simulink model "speechCommandRecognition"  (R2021a)
settings: Solver=FixedStepDiscrete  StartTime=0.0  StopTime=inf  RelTol=1e-3
InitFcn:
  | % Specify the audio sampling rate and classification rate in Hz and create
  | % an audio device reader that can read audio from your microphone.
  | fs = 16e3;
  | classificationRate = 10;
  | epsil = 1e-6;
  | numBands = 40;
  | 
  | % Audio device samples per frame
  | samplesPerFrame = floor(fs/classificationRate);
  | 
  | % Specify frameDuration and hopDuration for the melSpectrogram (in seconds)
  | frameDuration = 0.025;
  | hopDuration = 0.01;
  | 
  | % Frame and hop length for melSpectrogram in samples
  | frameLength = frameDuration*fs;
  | hopLength = hopDuration*fs;
  | 
  | % Spectrogram width (in time)
  | specWidthTime = 1 * fs;
  | 
  | % Spectrogram width (in samples)
  | specWidth = floor((specWidthTime-frameLength) / hopLength) + 1;
libraries: dspvision x3, audiosources x1, deeplib x1, simulink x1
settings Model: Creator=The MathWorks, Inc.  LastModifiedBy=The MathWorks, Inc.
settings SolverCC: AlgebraicLoopSolver=TrustRegion  AutoInsertRateTranBlk=on
settings DataIOCC: LimitDataPoints=on  SaveOutput=off  SignalLogging=off  SaveTime=off
settings OptimizationCC: LifeSpan=inf  SimCompilerOptimization=on
settings DebuggingCC: AlgebraicLoopMsg=error  SingleTaskRateTransMsg=error  IntegerOverflowMsg=none  AllowSymbolicDim=off  SFUnexpectedBacktrackingDiag=warning  SFNoUnconditionalDefaultTransitionDiag=warning  SFExecutionAtInitializationDiag=none  SFMachineParentedDataDiag=warning  IntegerSaturationMsg=none  ArithmeticOperatorsInVariantConditions=warning
settings SFSimCC: SimCtrlC=off  SimUseLocalCustomCode=off  CustomCodeUndefinedFunction=UseInterfaceOnly
settings RTWCC: RTWUseLocalCustomCode=off
settings CodeAppCC: StateflowObjectComments=on
settings GRTTargetCC: TargetLangStandard=C89/C90 (ANSI)
settings ConfigComp: CovMetricSettings=dw  CovSaveCumulativeToWorkspaceVar=on  CovSaveSingleToWorkspaceVar=on  CovExternalEMLEnable=off  CovSFcnEnable=off

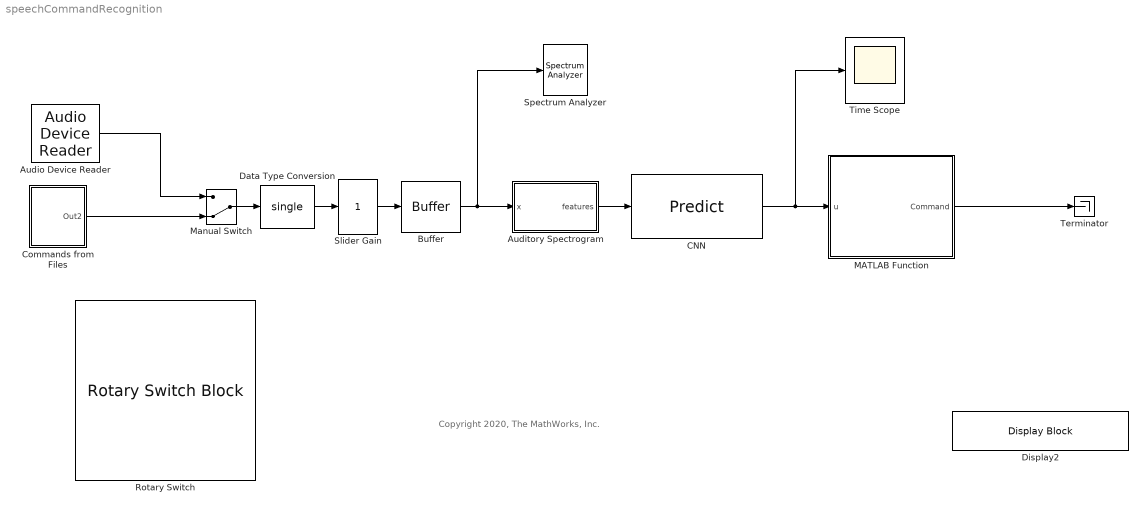
== system speechCommandRecognition ==
  note: Copyright 2020, The MathWorks, Inc.
  Audio Device Reader : audiosources/Audio Device Reader  Driver=CoreAudio  Device=No audio input device detected  SampleRate=fs  NumChannels=1  SamplesPerFrame=samplesPerFrame  BitDepth=16-bit integer  NumBuffers=10  DefaultInputChannelMapping=on  InputChannelMapping=1:2  OutputNumOverrunSamples=off  OutputDataType=double  DriverIdx=5  DeviceWarnFlag=''
      settings: SourceProductBaseCode=AU
  Auditory Spectrogram : MATLAB Function  TreatAsAtomicUnit=on
  Buffer : Buffer  N=fs  V=fs - samplesPerFrame  OutputFrames=off
  CNN : deeplib/Predict  Network=Network from MAT-file  NetworkFunction=squeezenet  NetworkFilePath=commandNet.mat  MiniBatchSize=1  InputDataFormats={ '', '' }  Predictions=off  Activations={ 'softmax' }  ForceInterpretedSim=off  EnableDLNetwork=off
      settings: SourceProductBaseCode=NN
  Commands from Files : Subsystem
  Data Type Conversion : DataTypeConversion  OutDataTypeStr=single
  Display2 : DisplayBlock  LabelPosition=Hide  Format=short
  MATLAB Function : MATLAB Function  TreatAsAtomicUnit=on
  Manual Switch : ManualSwitch  CurrentSetting=0
  Rotary Switch : RotarySwitchBlock
      settings: Values={{'Go', 'Yes', 'Stop'}, [1 2 3]}
  Slider Gain : simulink/Math Operations/Slider Gain  gain=1  low=0  high=30
  Spectrum Analyzer : SpectrumAnalyzer
  Terminator : Terminator
  Time Scope : Scope
  wires:
  Manual Switch/1 -> Data Type Conversion/1
  MATLAB Function/1(Command) -> Terminator/1
  Auditory Spectrogram/1(features) -> CNN/1
  Slider Gain/1 -> Buffer/1
  CNN/1 -> MATLAB Function/1(u), Time Scope/1
  Buffer/1 -> Auditory Spectrogram/1(x), Spectrum Analyzer/1
  Data Type Conversion/1 -> Slider Gain/1
  Commands from Files/1(Out2) -> Manual Switch/2
  Audio Device Reader/1 -> Manual Switch/1

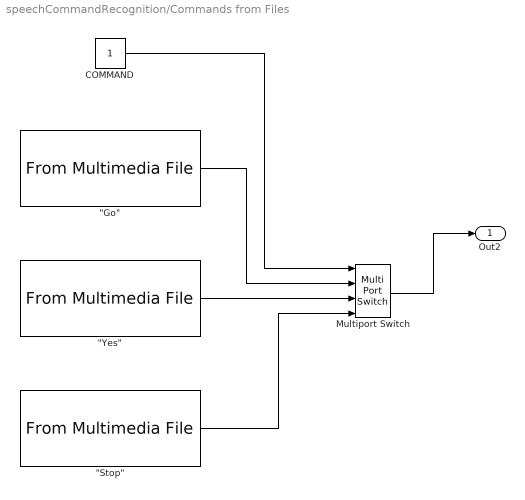
== system speechCommandRecognition/Commands from Files ==
  " \"Stop\"" : dspvision/From Multimedia File  inputFilename=stopCommand.flac  readRange=[1 Inf]  loop=on  numPlays=inf  outputStreams=Audio only  videoDataType=single  audioDataType=double  inheritSampleTime=on  userDefinedSampleTime=1/30  noAudioOutput=off  isIntensityVideo=off  fourcc=RGB  colorVideoFormat=Separate color signals  outputEOF=off  dataOrg=Column-major  audioFrameSize=samplesPerFrame  computeAudioFrameSize=off  outSamplingMode=Sample based
  "\"Go\"" : dspvision/From Multimedia File  inputFilename=goCommand.flac  readRange=[1 Inf]  loop=on  numPlays=inf  outputStreams=Audio only  videoDataType=single  audioDataType=double  inheritSampleTime=on  userDefinedSampleTime=1/30  noAudioOutput=off  isIntensityVideo=off  fourcc=RGB  colorVideoFormat=Separate color signals  outputEOF=off  dataOrg=Column-major  audioFrameSize=samplesPerFrame  computeAudioFrameSize=off  outSamplingMode=Sample based
  "\"Yes\"" : dspvision/From Multimedia File  inputFilename=yesCommand.flac  readRange=[1 Inf]  loop=on  numPlays=inf  outputStreams=Audio only  videoDataType=single  audioDataType=double  inheritSampleTime=on  userDefinedSampleTime=1/30  noAudioOutput=off  isIntensityVideo=off  fourcc=RGB  colorVideoFormat=Separate color signals  outputEOF=off  dataOrg=Column-major  audioFrameSize=samplesPerFrame  computeAudioFrameSize=off  outSamplingMode=Sample based
  COMMAND : Constant
  Multiport Switch : MultiPortSwitch
  Out2 : Outport
  wires:
  "\"Yes\""/1 -> Multiport Switch/3
  " \"Stop\""/1 -> Multiport Switch/4
  Multiport Switch/1 -> Out2/1
  "\"Go\""/1 -> Multiport Switch/2
  COMMAND/1 -> Multiport Switch/1

== matlab function speechCommandRecognition/MATLAB Function ==
  data: u input; classificationRate parameter; Command output size=[1 1]
function Command = postProcess(u,classificationRate)

    persistent YBuffer probBuffer
    
    if(isempty(YBuffer))
        YBuffer = ones(classificationRate,1);
        probBuffer = zeros([numel(u),round(classificationRate/2)]);
        prevCommand = SpeechCommands(0);
    end
    
    % Input u is array of 12 probability values (which word was most likely
    % to be spoken)

    % Find index of array with highest probability and enumerate to our
    % word
    [~,YPredicted] = max(u);
    
    % Add to buffers
    YBuffer(1:end-1)= YBuffer(2:end);
    YBuffer(end) = YPredicted;
    probBuffer(:,1:end-1) = probBuffer(:,2:end);
    probBuffer(:,end) = u;
    
    % Now do the actual command detection by performing a very simple
    % thresholding operation. Declare a detection and display it 
    % if all of the following hold:
    % 1) The most common label is not |background|.
    % 2) At least |countThreshold| of the latest frame labels agree.
    % 3) The maximum predicted probability of the predicted label is at
    % least |probThreshold|. Otherwise, do not declare a detection.

    [YMode,count] = mode(YBuffer,1);
    countThreshold = ceil(classificationRate*0.2);
    maxProb = max(probBuffer(YMode,:));
    probThreshold = 0.5;

    if (count > countThreshold && maxProb > probThreshold && YMode ~= SpeechCommands.Background)
        Command = SpeechCommands(YMode);
        prevCommand = Command;
    else
        Command = SpeechCommands(0);
    end
    
end

== matlab function speechCommandRecognition/Auditory Spectrogram ==
  data: x input size=[specWidthTime 1]; features output size=[98 50]
function features = fcn(x)

features = extractSpeechFeatures(x);
epsil = 1e-6;
features = log10(features + epsil);
